simulink model "HW6prob2b"  (Simulink 7.8)
settings: Solver=ode45  StartTime=0.0  StopTime=6  RelTol=1e-3
values from neighbouring files (symbols this model uses):
  A = [0, 1; -2, -3]    [16-31-hw-6.m]
  B = [0; 1]    [16-31-hw-6.m]
  K = Kb    [16-31-hw-6.m]
  Nbarb = 0.5*(1-K(2))-(1-K(1))    [16-31-hw-6.m]
  uncert = 0.1    [16-31-hw-6.m]
settings Model: Creator=Dan  LastModifiedBy=Dan

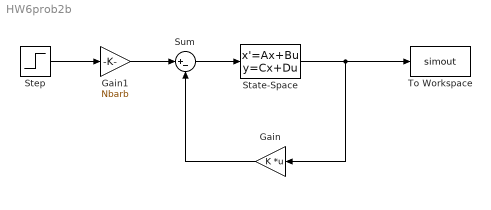
== system HW6prob2b ==
  Gain : Gain  Gain=K  Multiplication=Matrix(K*u)
  Gain1 : Gain  Gain=Nbarb
  State-Space : StateSpace  A=A+eye(2,2)*uncert  B=B  C=eye(2,2)  D=[0;0]
  Step : Step  SampleTime=0
  Sum : Sum  Inputs=|+-
  To Workspace : ToWorkspace  VariableName=simout  SampleTime=-1  SaveFormat=Structure
  wires:
  Gain/1 -> Sum/2
  Sum/1 -> State-Space/1
  State-Space/1 -> Gain/1, To Workspace/1
  Step/1 -> Gain1/1
  Gain1/1 -> Sum/1
